simulink model "MainSystem"  (R2020b)
settings: Solver=VariableStepAuto  StartTime=0.0  StopTime=5000  RelTol=1e-3
libraries: pid_lib x1
settings Model: Creator=BALUCH  LastModifiedBy=BALUCH

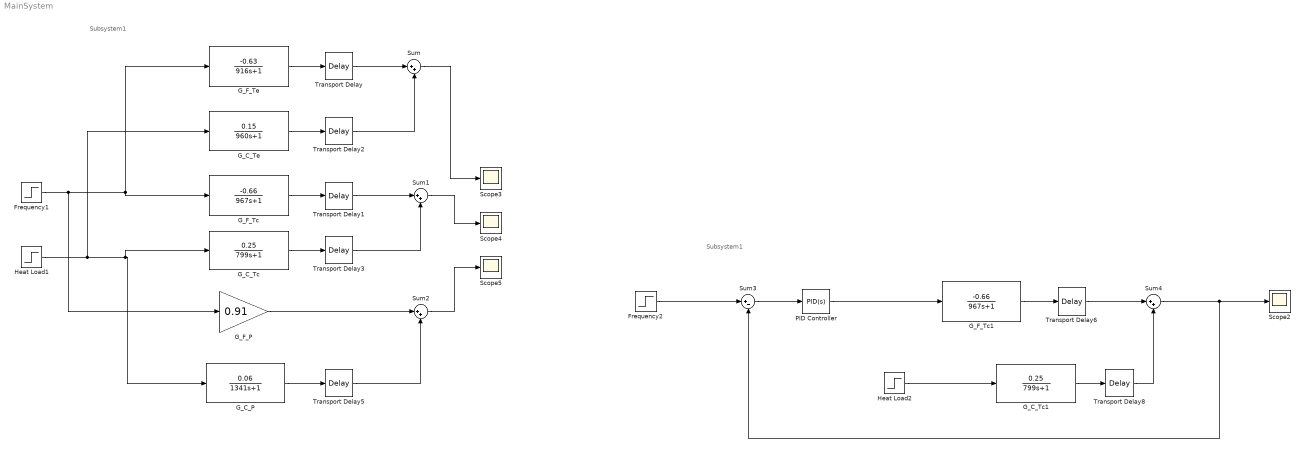
== system MainSystem ==
  note: Subsystem1
  note: Subsystem1
  Frequency1 : Step  Time=60  SampleTime=0
  Frequency2 : Step  Time=60  SampleTime=0
  G_C_P : TransferFcn  Numerator=[0.06]  Denominator=[1341 1]
  G_C_Tc : TransferFcn  Numerator=[0.25]  Denominator=[799 1]
  G_C_Tc1 : TransferFcn  Numerator=[0.25]  Denominator=[799 1]
  G_C_Te : TransferFcn  Numerator=[0.15]  Denominator=[960 1]
  G_F_P : Gain  Gain=0.91
  G_F_Tc : TransferFcn  Numerator=[-0.66]  Denominator=[967 1]
  G_F_Tc1 : TransferFcn  Numerator=[-0.66]  Denominator=[967 1]
  G_F_Te : TransferFcn  Numerator=[-0.63]  Denominator=[916 1]
  Heat Load1 : Step  Time=10  SampleTime=0
  Heat Load2 : Step  Time=1430  SampleTime=0
  PID Controller : pid_lib/PID Controller  Controller=PID  Form=Parallel  TimeDomain=Continuous-time  UseExternalTs=off  SampleTime=-1  IntegratorMethod=Forward Euler  FilterMethod=Forward Euler  ControllerParametersSource=internal  P=1  I=1  D=0  UseFilter=on  N=100  TunerSelectOption=Transfer Function Based (PID Tuner App)  InitialConditionSource=internal  InitialConditionForIntegrator=0  InitialConditionForFilter=0  DifferentiatorICPrevScaledInput=0  ExternalReset=none  TrackingMode=off  Kt=1  LimitOutput=off  SatLimitsSource=internal  UpperSaturationLimit=inf  LowerSaturationLimit=-inf  LinearizeAsGain=on  AntiWindupMode=none  Kb=1  POutMin=[]  POutMax=[]  IOutMin=[]  IOutMax=[]  DOutMin=[]  DOutMax=[]  NOutMin=[]  NOutMax=[]  SumOutMin=[]  SumOutMax=[]  SaturationOutMin=[]  SaturationOutMax=[]  PParamMin=[]  PParamMax=[]  IParamMin=[]  IParamMax=[]  DParamMin=[]  DParamMax=[]  NParamMin=[]  NParamMax=[]  KbParamMin=[]  KbParamMax=[]  KtParamMin=[]  KtParamMax=[]  KbOutMin=[]  KbOutMax=[]  KtOutMin=[]  KtOutMax=[]  IntegratorOutMin=[]  IntegratorOutMax=[]  FilterOutMin=[]  FilterOutMax=[]  SumI1OutMin=[]  SumI1OutMax=[]  SumI2OutMin=[]  SumI2OutMax=[]  SumI3OutMin=[]  SumI3OutMax=[]  SumI4OutMin=[]  SumI4OutMax=[]  SumDOutMin=[]  SumDOutMax=[]  DifferentiatorOutMin=[]  DifferentiatorOutMax=[]  FilterDiffOutCoefMin=[]  FilterDiffOutCoefMax=[]  ReciprocalOutMin=[]  ReciprocalOutMax=[]  SumDenOutMin=[]  SumDenOutMax=[]  SumNumOutMin=[]  SumNumOutMax=[]  DivideOutMin=[]  DivideOutMax=[]  UdiffTsProdOutMin=[]  UdiffTsProdOutMax=[]  NTsProdOutMin=[]  NTsProdOutMax=[]  UintegralTsProdOutMin=[]  UintegralTsProdOutMax=[]  UngainTsProdOutMin=[]  UngainTsProdOutMax=[]  IntegratorContinuousStateAttributes=''  IntegratorStateMustResolveToSignalObject=off  IntegratorRTWStateStorageClass=Auto  FilterContinuousStateAttributes=''  FilterStateMustResolveToSignalObject=off  FilterRTWStateStorageClass=Auto  ParallelPVariant=InternalParameters  IdealPVariant=Disabled  IVariant=InternalParameters  DVariant=InternalParameters  IntegratorVariant=Continuous  SatVariant=Disabled  AWVariant=Passthrough  PCopyVariant=Disabled  TRVariant=Disabled  FdbkBlocksVariant=Forward  IdealPFdbkVariant=Disabled  SatFdbkVariant=Disabled  DerivativeFilterVariant=ContFilter  NVariant=InternalParameters  NCopyVariant=Disabled  FilterICVariant=InternalICsFilter  IntegratorICVariant=InternalICs  ExternalResetVariant=Disabled  TRSumVariant=Passthrough  SumFdbkVariant=Disabled  SumVariant=Sum_PID  TsampFilterVariant=InternalTs  TsampNgainVariant=Passthrough  TsampIntegralVariant=Passthrough  ExternalSaturationOutDataTypeStr=Inherit: Same as second input
  Scope{2..5} (4 alike) : Scope
  Sum{,1..2,4} (4 alike) : Sum  Inputs=|++
  Sum3 : Sum  Inputs=|+-
  Transport Delay : TransportDelay  DelayTime=15
  Transport Delay1 : TransportDelay  DelayTime=35
  Transport Delay2 : TransportDelay  DelayTime=42
  Transport Delay3 : TransportDelay  DelayTime=15
  Transport Delay5 : TransportDelay  DelayTime=182
  Transport Delay6 : TransportDelay  DelayTime=35
  Transport Delay8 : TransportDelay  DelayTime=15
  wires:
  Sum2/1 -> Scope5/1
  Sum/1 -> Scope3/1
  Sum1/1 -> Scope4/1
  G_C_Tc/1 -> Transport Delay3/1
  G_C_P/1 -> Transport Delay5/1
  G_F_P/1 -> Sum2/1
  Transport Delay5/1 -> Sum2/2
  G_F_Tc/1 -> Transport Delay1/1
  Transport Delay3/1 -> Sum1/2
  G_C_Te/1 -> Transport Delay2/1
  Heat Load1/1 -> G_C_P/1, G_C_Tc/1, G_C_Te/1
  Transport Delay1/1 -> Sum1/1
  Frequency1/1 -> G_F_Tc/1, G_F_Te/1, G_F_P/1
  Transport Delay2/1 -> Sum/2
  Transport Delay/1 -> Sum/1
  G_F_Te/1 -> Transport Delay/1
  Transport Delay8/1 -> Sum4/2
  G_C_Tc1/1 -> Transport Delay8/1
  Sum4/1 -> Sum3/2, Scope2/1
  G_F_Tc1/1 -> Transport Delay6/1
  Transport Delay6/1 -> Sum4/1
  Heat Load2/1 -> G_C_Tc1/1
  Sum3/1 -> PID Controller/1
  PID Controller/1 -> G_F_Tc1/1
  Frequency2/1 -> Sum3/1
